simulink library "M160_lib"  (Simulink 7.8)
settings: Solver=FixedStepDiscrete  StartTime=0.0  StopTime=10.0  RelTol=1e-3
PreLoadFcn:
  | update_path
undefined symbols (not defined in the file): Afr_atCool2facLambdaReqCorr_CUR_x, Afr_atCool2facLambdaReqCorr_CUR_y, Afr_atMani2facLambdaReqCorr_CUR_x, Afr_atMani2facLambdaReqCorr_CUR_y, Afr_facLambdaReqMan, Afr_facRatioMan, Afr_facStoich, Afr_flgLambdaReqOverride, Afr_flgRatioOverride, Afr_rpmEngSpdfacRelAir2facLambdaReqBase_MAP_x, Afr_rpmEngSpdfacRelAir2facLambdaReqBase_MAP_y, Afr_rpmEngSpdfacRelAir2facLambdaReqBase_MAP_z, Ais_flgAirInjReacPumpOverride, Ais_stAirInjReacPumpMan, Amc_flgAirMassFlowOverride, Amc_uSens2AirMassFlow_CUR_x, Amc_uSens2AirMassFlow_CUR_y, Amc_uSensMaxValid, Amc_uSensMinValid, Amf_facRelAirMan, Amf_flgAirMassPerStrOverride, Amf_flgRelAirOverride, Amf_flgSwitch2AirMassFlowMeter, Amf_mAirPerStrMan, Amf_pManiEngSpd2facRelAirCorr_MAP_x, Amf_pManiEngSpd2facRelAirCorr_MAP_y, Amf_pManiEngSpd2facRelAirCorr_MAP_z, Amf_rpmEngSpd2facTempCorr_CUR_x, Amf_rpmEngSpd2facTempCorr_CUR_y, Amf_shcSpecGasConst_C, Amf_volEngDisp_C, Apv_facAirPumpRateMan, Apv_factor, Apv_flgAirPumpRateOverride, Apv_tiPeriod_C, Bvc_rVoltDivHigh, Bvc_rVoltDivLow, Bvc_uBattMax, Bvc_uBattMin, CDRV_E_OK_, Cov_facChOverVlvRateMan, Cov_factor, Cov_flgChOverVlvRateOverride, Cov_tiPeriod_C, Cpc_atManiTmp2facPresCorr_CUR_x, Cpc_atManiTmp2facPresCorr_CUR_y, Cpc_flgPChargeOverride, Cpc_uSens2pManiBase_CUR_x, Cpc_uSens2pManiBase_CUR_y, Ctc_rPullUp_C, Ctc_rSens2atCool_CUR_x, Ctc_rSens2atCool_CUR_y, Ctc_uSensMaxValid, Ctc_uSensMinValid, Ctc_uSupply, Doh_OutputDiagnosisOverride, dummy_facAirPumpRateReq, dummy_facChOverVlvRateReq, dummy_flgInterCoolerOverride, dummy_flgKl50Override ... (+243)
libraries: simulink x36, ehooks_lib x3
(part 6 of 8)

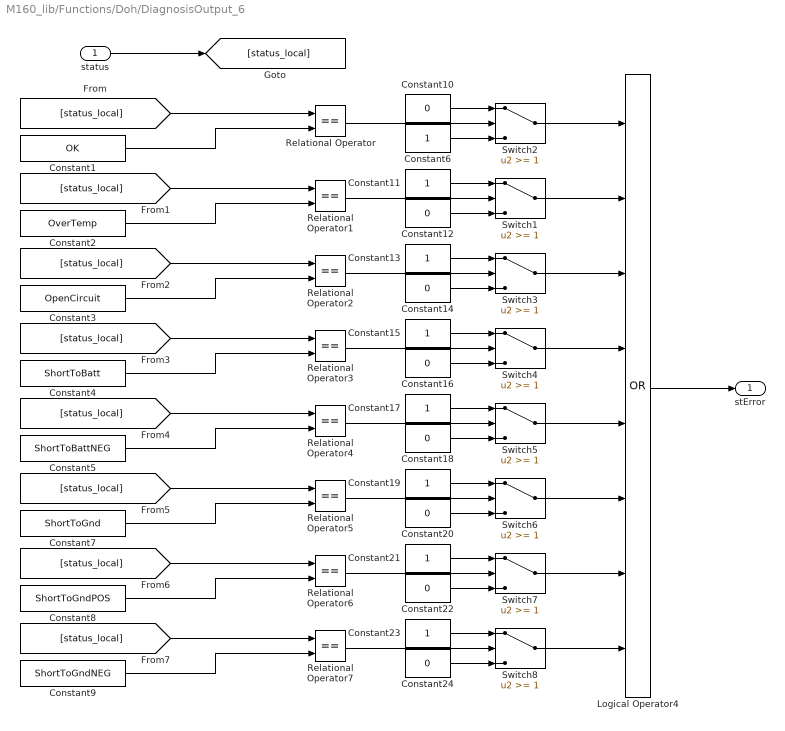
== system M160_lib/Functions/Doh/DiagnosisOutput_6 ==
  status : Inport
  Constant1 : Constant  Value=OK
  Constant{10,12,14,16,18,20,22,24} (8 alike) : Constant  Value=0  OutDataTypeStr=boolean
  Constant{6,11,13,15,17,19,21,23} (8 alike) : Constant  OutDataTypeStr=boolean
  Constant2 : Constant  Value=OverTemp
  Constant3 : Constant  Value=OpenCircuit
  Constant4 : Constant  Value=ShortToBatt
  Constant5 : Constant  Value=ShortToBattNEG
  Constant7 : Constant  Value=ShortToGnd
  Constant8 : Constant  Value=ShortToGndPOS
  Constant9 : Constant  Value=ShortToGndNEG
  Logical Operator4 : Logic  Operator=OR  Inputs=8  AllPortsSameDT=off  OutDataTypeStr=boolean
  Relational Operator{,1..7} (8 alike) : RelationalOperator  Operator===  OutDataTypeStr=boolean
  Switch{1..8} (8 alike) : Switch  Threshold=1
  stError : Outport
  wires:
  Switch8/1 -> Logical Operator4/8
  Switch7/1 -> Logical Operator4/7
  Switch6/1 -> Logical Operator4/6
  Switch5/1 -> Logical Operator4/5
  Switch4/1 -> Logical Operator4/4
  Switch3/1 -> Logical Operator4/3
  Switch1/1 -> Logical Operator4/2
  Switch2/1 -> Logical Operator4/1
  Relational Operator7/1 -> Switch8/2
  Constant23/1 -> Switch8/1
  Constant24/1 -> Switch8/3
  Relational Operator6/1 -> Switch7/2
  Constant21/1 -> Switch7/1
  Constant22/1 -> Switch7/3
  Relational Operator5/1 -> Switch6/2
  Constant19/1 -> Switch6/1
  Constant20/1 -> Switch6/3
  Relational Operator4/1 -> Switch5/2
  Constant17/1 -> Switch5/1
  Constant18/1 -> Switch5/3
  Relational Operator3/1 -> Switch4/2
  Constant15/1 -> Switch4/1
  Constant16/1 -> Switch4/3
  Relational Operator2/1 -> Switch3/2
  Constant13/1 -> Switch3/1
  Constant14/1 -> Switch3/3
  Relational Operator1/1 -> Switch1/2
  Constant11/1 -> Switch1/1
  Constant12/1 -> Switch1/3
  Constant10/1 -> Switch2/1
  Logical Operator4/1 -> stError/1
  Constant6/1 -> Switch2/3
  Relational Operator/1 -> Switch2/2
  [status_local] -> Relational Operator7/1
  Constant9/1 -> Relational Operator7/2
  [status_local] -> Relational Operator6/1
  Constant8/1 -> Relational Operator6/2
  [status_local] -> Relational Operator5/1
  Constant7/1 -> Relational Operator5/2
  [status_local] -> Relational Operator4/1
  Constant5/1 -> Relational Operator4/2
  [status_local] -> Relational Operator3/1
  Constant4/1 -> Relational Operator3/2
  [status_local] -> Relational Operator2/1
  Constant3/1 -> Relational Operator2/2
  [status_local] -> Relational Operator1/1
  Constant2/1 -> Relational Operator1/2
  [status_local] -> Relational Operator/1
  status/1 -> [status_local]
  Constant1/1 -> Relational Operator/2

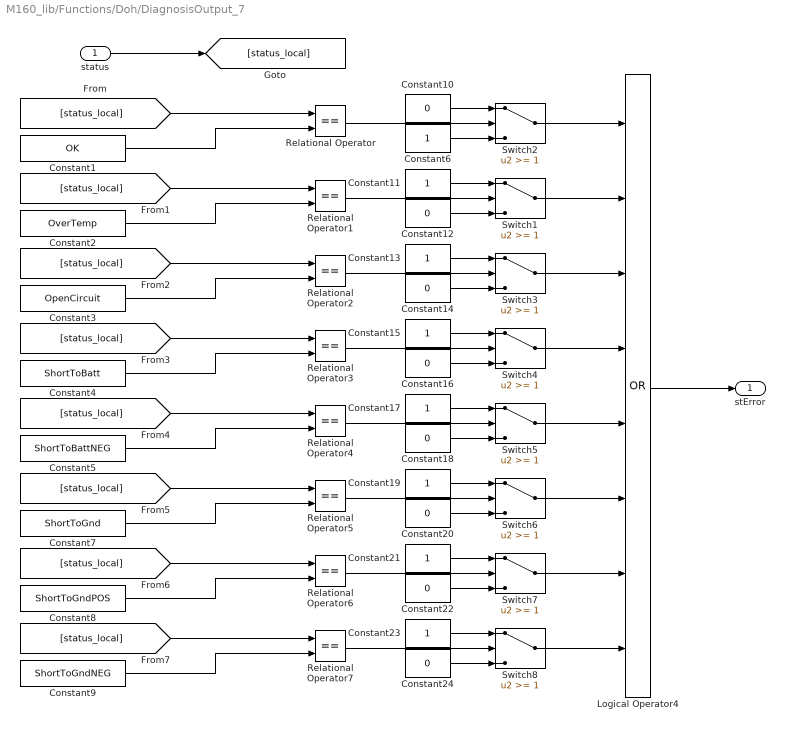
== system M160_lib/Functions/Doh/DiagnosisOutput_7 ==
  status : Inport
  Constant1 : Constant  Value=OK
  Constant{10,12,14,16,18,20,22,24} (8 alike) : Constant  Value=0  OutDataTypeStr=boolean
  Constant{6,11,13,15,17,19,21,23} (8 alike) : Constant  OutDataTypeStr=boolean
  Constant2 : Constant  Value=OverTemp
  Constant3 : Constant  Value=OpenCircuit
  Constant4 : Constant  Value=ShortToBatt
  Constant5 : Constant  Value=ShortToBattNEG
  Constant7 : Constant  Value=ShortToGnd
  Constant8 : Constant  Value=ShortToGndPOS
  Constant9 : Constant  Value=ShortToGndNEG
  Logical Operator4 : Logic  Operator=OR  Inputs=8  AllPortsSameDT=off  OutDataTypeStr=boolean
  Relational Operator{,1..7} (8 alike) : RelationalOperator  Operator===  OutDataTypeStr=boolean
  Switch{1..8} (8 alike) : Switch  Threshold=1
  stError : Outport
  wires:
  Constant1/1 -> Relational Operator/2
  status/1 -> [status_local]
  [status_local] -> Relational Operator/1
  Constant2/1 -> Relational Operator1/2
  [status_local] -> Relational Operator1/1
  Constant3/1 -> Relational Operator2/2
  [status_local] -> Relational Operator2/1
  Constant4/1 -> Relational Operator3/2
  [status_local] -> Relational Operator3/1
  Constant5/1 -> Relational Operator4/2
  [status_local] -> Relational Operator4/1
  Constant7/1 -> Relational Operator5/2
  [status_local] -> Relational Operator5/1
  Constant8/1 -> Relational Operator6/2
  [status_local] -> Relational Operator6/1
  Constant9/1 -> Relational Operator7/2
  [status_local] -> Relational Operator7/1
  Relational Operator/1 -> Switch2/2
  Constant6/1 -> Switch2/3
  Logical Operator4/1 -> stError/1
  Constant10/1 -> Switch2/1
  Constant12/1 -> Switch1/3
  Constant11/1 -> Switch1/1
  Relational Operator1/1 -> Switch1/2
  Constant14/1 -> Switch3/3
  Constant13/1 -> Switch3/1
  Relational Operator2/1 -> Switch3/2
  Constant16/1 -> Switch4/3
  Constant15/1 -> Switch4/1
  Relational Operator3/1 -> Switch4/2
  Constant18/1 -> Switch5/3
  Constant17/1 -> Switch5/1
  Relational Operator4/1 -> Switch5/2
  Constant20/1 -> Switch6/3
  Constant19/1 -> Switch6/1
  Relational Operator5/1 -> Switch6/2
  Constant22/1 -> Switch7/3
  Constant21/1 -> Switch7/1
  Relational Operator6/1 -> Switch7/2
  Constant24/1 -> Switch8/3
  Constant23/1 -> Switch8/1
  Relational Operator7/1 -> Switch8/2
  Switch2/1 -> Logical Operator4/1
  Switch1/1 -> Logical Operator4/2
  Switch3/1 -> Logical Operator4/3
  Switch4/1 -> Logical Operator4/4
  Switch5/1 -> Logical Operator4/5
  Switch6/1 -> Logical Operator4/6
  Switch7/1 -> Logical Operator4/7
  Switch8/1 -> Logical Operator4/8

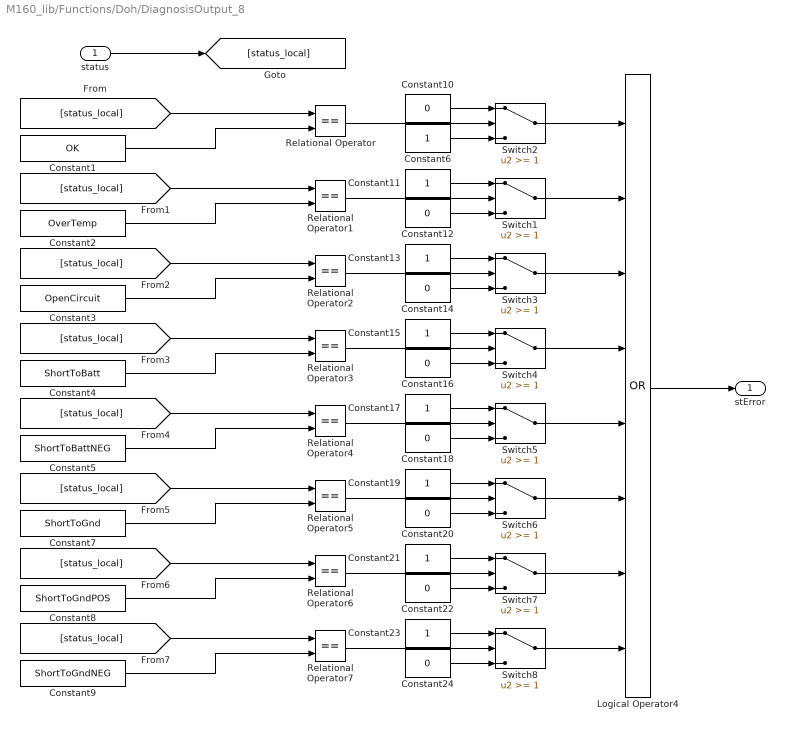
== system M160_lib/Functions/Doh/DiagnosisOutput_8 ==
  status : Inport
  Constant1 : Constant  Value=OK
  Constant{10,12,14,16,18,20,22,24} (8 alike) : Constant  Value=0  OutDataTypeStr=boolean
  Constant{6,11,13,15,17,19,21,23} (8 alike) : Constant  OutDataTypeStr=boolean
  Constant2 : Constant  Value=OverTemp
  Constant3 : Constant  Value=OpenCircuit
  Constant4 : Constant  Value=ShortToBatt
  Constant5 : Constant  Value=ShortToBattNEG
  Constant7 : Constant  Value=ShortToGnd
  Constant8 : Constant  Value=ShortToGndPOS
  Constant9 : Constant  Value=ShortToGndNEG
  Logical Operator4 : Logic  Operator=OR  Inputs=8  AllPortsSameDT=off  OutDataTypeStr=boolean
  Relational Operator{,1..7} (8 alike) : RelationalOperator  Operator===  OutDataTypeStr=boolean
  Switch{1..8} (8 alike) : Switch  Threshold=1
  stError : Outport
  wires:
  Switch8/1 -> Logical Operator4/8
  Switch7/1 -> Logical Operator4/7
  Switch6/1 -> Logical Operator4/6
  Switch5/1 -> Logical Operator4/5
  Switch4/1 -> Logical Operator4/4
  Switch3/1 -> Logical Operator4/3
  Switch1/1 -> Logical Operator4/2
  Switch2/1 -> Logical Operator4/1
  Relational Operator7/1 -> Switch8/2
  Constant23/1 -> Switch8/1
  Constant24/1 -> Switch8/3
  Relational Operator6/1 -> Switch7/2
  Constant21/1 -> Switch7/1
  Constant22/1 -> Switch7/3
  Relational Operator5/1 -> Switch6/2
  Constant19/1 -> Switch6/1
  Constant20/1 -> Switch6/3
  Relational Operator4/1 -> Switch5/2
  Constant17/1 -> Switch5/1
  Constant18/1 -> Switch5/3
  Relational Operator3/1 -> Switch4/2
  Constant15/1 -> Switch4/1
  Constant16/1 -> Switch4/3
  Relational Operator2/1 -> Switch3/2
  Constant13/1 -> Switch3/1
  Constant14/1 -> Switch3/3
  Relational Operator1/1 -> Switch1/2
  Constant11/1 -> Switch1/1
  Constant12/1 -> Switch1/3
  Constant10/1 -> Switch2/1
  Logical Operator4/1 -> stError/1
  Constant6/1 -> Switch2/3
  Relational Operator/1 -> Switch2/2
  [status_local] -> Relational Operator7/1
  Constant9/1 -> Relational Operator7/2
  [status_local] -> Relational Operator6/1
  Constant8/1 -> Relational Operator6/2
  [status_local] -> Relational Operator5/1
  Constant7/1 -> Relational Operator5/2
  [status_local] -> Relational Operator4/1
  Constant5/1 -> Relational Operator4/2
  [status_local] -> Relational Operator3/1
  Constant4/1 -> Relational Operator3/2
  [status_local] -> Relational Operator2/1
  Constant3/1 -> Relational Operator2/2
  [status_local] -> Relational Operator1/1
  Constant2/1 -> Relational Operator1/2
  [status_local] -> Relational Operator/1
  status/1 -> [status_local]
  Constant1/1 -> Relational Operator/2

== system M160_lib/Functions/Doh/DiagnosisOutput_9 ==
  status : Inport
  Constant1 : Constant  Value=OK
  Constant{10,12,14,16,18,20,22,24} (8 alike) : Constant  Value=0  OutDataTypeStr=boolean
  Constant{6,11,13,15,17,19,21,23} (8 alike) : Constant  OutDataTypeStr=boolean
  Constant2 : Constant  Value=OverTemp
  Constant3 : Constant  Value=OpenCircuit
  Constant4 : Constant  Value=ShortToBatt
  Constant5 : Constant  Value=ShortToBattNEG
  Constant7 : Constant  Value=ShortToGnd
  Constant8 : Constant  Value=ShortToGndPOS
  Constant9 : Constant  Value=ShortToGndNEG
  Logical Operator4 : Logic  Operator=OR  Inputs=8  AllPortsSameDT=off  OutDataTypeStr=boolean
  Relational Operator{,1..7} (8 alike) : RelationalOperator  Operator===  OutDataTypeStr=boolean
  Switch{1..8} (8 alike) : Switch  Threshold=1
  stError : Outport
  wires:
  Constant1/1 -> Relational Operator/2
  status/1 -> [status_local]
  [status_local] -> Relational Operator/1
  Constant2/1 -> Relational Operator1/2
  [status_local] -> Relational Operator1/1
  Constant3/1 -> Relational Operator2/2
  [status_local] -> Relational Operator2/1
  Constant4/1 -> Relational Operator3/2
  [status_local] -> Relational Operator3/1
  Constant5/1 -> Relational Operator4/2
  [status_local] -> Relational Operator4/1
  Constant7/1 -> Relational Operator5/2
  [status_local] -> Relational Operator5/1
  Constant8/1 -> Relational Operator6/2
  [status_local] -> Relational Operator6/1
  Constant9/1 -> Relational Operator7/2
  [status_local] -> Relational Operator7/1
  Relational Operator/1 -> Switch2/2
  Constant6/1 -> Switch2/3
  Logical Operator4/1 -> stError/1
  Constant10/1 -> Switch2/1
  Constant12/1 -> Switch1/3
  Constant11/1 -> Switch1/1
  Relational Operator1/1 -> Switch1/2
  Constant14/1 -> Switch3/3
  Constant13/1 -> Switch3/1
  Relational Operator2/1 -> Switch3/2
  Constant16/1 -> Switch4/3
  Constant15/1 -> Switch4/1
  Relational Operator3/1 -> Switch4/2
  Constant18/1 -> Switch5/3
  Constant17/1 -> Switch5/1
  Relational Operator4/1 -> Switch5/2
  Constant20/1 -> Switch6/3
  Constant19/1 -> Switch6/1
  Relational Operator5/1 -> Switch6/2
  Constant22/1 -> Switch7/3
  Constant21/1 -> Switch7/1
  Relational Operator6/1 -> Switch7/2
  Constant24/1 -> Switch8/3
  Constant23/1 -> Switch8/1
  Relational Operator7/1 -> Switch8/2
  Switch2/1 -> Logical Operator4/1
  Switch1/1 -> Logical Operator4/2
  Switch3/1 -> Logical Operator4/3
  Switch4/1 -> Logical Operator4/4
  Switch5/1 -> Logical Operator4/5
  Switch6/1 -> Logical Operator4/6
  Switch7/1 -> Logical Operator4/7
  Switch8/1 -> Logical Operator4/8

== system M160_lib/Functions/Fmc/DT1 ==
  T : Inport
  K : Inport  Port=2
  Ta : Inport  Port=3
  in : Inport  Port=4
  initValue : Inport  Port=5
  Enable : Inport  Port=6
  Add2 : Sum  OutDataTypeStr=Inherit: Same as first input
  Constan3 : Constant  OutDataTypeStr=single
  Divide1 : Product  Inputs=*/  OutDataTypeStr=Inherit: Same as first input
  Product1 : Product  Inputs=3  OutDataTypeStr=Inherit: Same as first input
  Product3 : Product  OutDataTypeStr=Inherit: Same as first input
  Product4 : Product  OutDataTypeStr=Inherit: Same as first input
  Subtract1 : Sum  Inputs=+-
  Switch1 : Switch  Threshold=1
  Unit Delay4 : UnitDelay  SampleTime=-1
  Unit Delay5 : UnitDelay  SampleTime=-1
  Unit Delay6 : UnitDelay  SampleTime=-1
  Out : Outport
  wires:
  initValue/1 -> Switch1/3
  Switch1/1 -> Out/1
  in/1 -> Subtract1/1
  Subtract1/1 -> Product3/2
  K/1 -> Product3/1, Product4/2
  Product3/1 -> Unit Delay6/1
  Unit Delay6/1 -> Product1/1
  Constan3/1 -> Divide1/1
  T/1 -> Product4/1
  Product4/1 -> Divide1/2
  Divide1/1 -> Product1/2
  Product1/1 -> Add2/1
  Add2/1 -> Unit Delay5/1, Unit Delay4/1, Switch1/1
  Unit Delay5/1 -> Add2/2
  Unit Delay4/1 -> Subtract1/2
  Ta/1 -> Product1/3
  Enable/1 -> Switch1/2

== system M160_lib/Functions/Fmc/DT1_Fcn ==
  In : Inport
  initValue : Inport  Port=2
  Enable : Inport  Port=3
  Discrete Transfer Fcn : DiscreteTransferFcn  Numerator=[Fmc_facKFuelMassCorr Fmc_facKFuelMassCorr*(0.001/Fmc_tiTFuelMassCorr-1)]  Denominator=[1 -1]  SampleTime=-1  OutDataTypeStr=Inherit: Same as input
  Switch1 : Switch  Threshold=1
  Out : Outport
  wires:
  In/1 -> Discrete Transfer Fcn/1
  initValue/1 -> Switch1/3
  Switch1/1 -> Out/1
  Discrete Transfer Fcn/1 -> Switch1/1
  Enable/1 -> Switch1/2

== system M160_lib/Functions/ICC_1/RSFlipFlop ==
  s : Inport
  r : Inport  Port=2
  Gain : Gain  OutDataTypeStr=Inherit: Same as input
  Logical Operator3 : Logic  Operator=NOT  AllPortsSameDT=off  OutDataTypeStr=boolean
  MATLAB Function : MATLAB Function  TreatAsAtomicUnit=on
  Unit Delay : UnitDelay  SampleTime=-1
  q : Outport
  nq : Outport  Port=2
  wires:
  Logical Operator3/1 -> nq/1
  r/1 -> MATLAB Function/1(r)
  s/1 -> MATLAB Function/2(s)
  MATLAB Function/1(q) -> Unit Delay/1
  Gain/1 -> q/1
  Unit Delay/1 -> Logical Operator3/1, Gain/1

== system M160_lib/Functions/Isc/CounterEnabled ==
  initEnable : Inport
  enable : Inport  Port=2
  Add1 : Sum
  Constant1 : Constant  OutDataTypeStr=single
  Constant2 : Constant  Value=0  OutDataTypeStr=single
  MATLAB Function : MATLAB Function  TreatAsAtomicUnit=on
  Switch2 : Switch  Threshold=1
  Unit Delay : UnitDelay  SampleTime=-1
  Unit Delay1 : UnitDelay  SampleTime=-1
  return : Outport
  wires:
  initEnable/1 -> MATLAB Function/1(u)
  MATLAB Function/1(y) -> Switch2/2
  Add1/1 -> Unit Delay1/1, Switch2/1
  Constant2/1 -> Switch2/3
  Switch2/1 -> Unit Delay/1
  Unit Delay1/1 -> Add1/2
  Constant1/1 -> Add1/1
  enable/1 -> MATLAB Function/2(v)
  Unit Delay/1 -> return/1

== system M160_lib/Functions/Isc/EdgeFalling ==
  signal : Inport
  Detect Decrease : simulink/Logic and Bit Operations/Detect Decrease  vinit=0.0  InputProcessing=Inherited  OutDataTypeStr=boolean
  return : Outport
  wires:
  Detect Decrease/1 -> return/1
  signal/1 -> Detect Decrease/1

== system M160_lib/Functions/Isc/EdgeRising ==
  signal : Inport
  Detect Increase : simulink/Logic and Bit Operations/Detect Increase  vinit=0.0  InputProcessing=Inherited  OutDataTypeStr=boolean
  return : Outport
  wires:
  Detect Increase/1 -> return/1
  signal/1 -> Detect Increase/1

== system M160_lib/Functions/Isc/Integrator ==
  initEnable : Inport
  enable : Inport  Port=2
  in : Inport  Port=3
  deltaT : Inport  Port=4
  mx : Inport  Port=5
  mn : Inport  Port=6
  initValue : Inport  Port=7
  Add : Sum
  MATLAB Function : MATLAB Function  TreatAsAtomicUnit=on
  MinMax : MinMax  Function=max  Inputs=2
  MinMax1 : MinMax  Inputs=2
  Product1 : Product  OutDataTypeStr=Inherit: Same as first input
  Unit Delay : UnitDelay  SampleTime=-1
  Unit Delay1 : UnitDelay  SampleTime=-1
  return : Outport
  wires:
  deltaT/1 -> Product1/2
  in/1 -> Product1/1
  Product1/1 -> Add/1
  Add/1 -> MinMax1/1
  mx/1 -> MinMax1/2
  MinMax1/1 -> MinMax/1
  mn/1 -> MinMax/2
  Unit Delay/1 -> Add/2
  MinMax/1 -> Unit Delay/1, MATLAB Function/4(in)
  MATLAB Function/1(out) -> Unit Delay1/1
  enable/1 -> MATLAB Function/3(enable)
  initValue/1 -> MATLAB Function/2(initValue)
  initEnable/1 -> MATLAB Function/1(initEnable)
  Unit Delay1/1 -> return/1

== system M160_lib/Functions/Isc/Integrator1 ==
  initEnable : Inport
  enable : Inport  Port=2
  in : Inport  Port=3
  deltaT : Inport  Port=4
  mx : Inport  Port=5
  mn : Inport  Port=6
  initValue : Inport  Port=7
  Add : Sum
  MATLAB Function : MATLAB Function  TreatAsAtomicUnit=on
  MinMax : MinMax  Function=max  Inputs=2
  MinMax1 : MinMax  Inputs=2
  Product1 : Product  OutDataTypeStr=Inherit: Same as first input
  Unit Delay : UnitDelay  SampleTime=-1
  Unit Delay1 : UnitDelay  SampleTime=-1
  return : Outport
  wires:
  Unit Delay1/1 -> return/1
  initEnable/1 -> MATLAB Function/1(initEnable)
  initValue/1 -> MATLAB Function/2(initValue)
  enable/1 -> MATLAB Function/3(enable)
  MATLAB Function/1(out) -> Unit Delay1/1
  MinMax/1 -> MATLAB Function/4(in), Unit Delay/1
  Unit Delay/1 -> Add/2
  mn/1 -> MinMax/2
  MinMax1/1 -> MinMax/1
  mx/1 -> MinMax1/2
  Add/1 -> MinMax1/1
  Product1/1 -> Add/1
  in/1 -> Product1/1
  deltaT/1 -> Product1/2

== system M160_lib/Functions/Itc/Hysteresis_Delta_RSP ==
  in : Inport
  Relay : Relay  OnSwitchValue=Itc_rpmEngSpdMax  OffSwitchValue=Itc_rpmEngSpdMax-Itc_rpmEngSpdHyst  OutDataTypeStr=Inherit: Inherit via back propagation
  return : Outport
  wires:
  Relay/1 -> return/1
  in/1 -> Relay/1

== system M160_lib/Functions/Lcc/PID-Controller ==
  in : Inport
  Lcc_flgSwitch2PIDController : Inport  Port=2
  dt : Inport  Port=3
  Lamsoni : Inport  Port=4
  Afr_facLambdaReq : Inport  Port=5
  Epm_rpmEngSpd : Inport  Port=6
  Mpc_pManiFilt : Inport  Port=7
  Constant8 : Constant  Value=Lcc_LambdaCorrMaxPID
  Constant9 : Constant  Value=Lcc_LambdaCorrMinPID
  Lcc_facKLambdaCorrPID_MAP : Lookup_n-D  BreakpointsForDimension1=Lcc_facKLambdaCorrPID_MAP_x  BreakpointsForDimension2=Lcc_facKLambdaCorrPID_MAP_y  Table=Lcc_facKLambdaCorrPID_MAP_z  ExtrapMethod=Clip  InputSameDT=on
  Lcc_tiTnLambdaCorrPID_MAP : Lookup_n-D  BreakpointsForDimension1=Lcc_tiTnLambdaCorrPID_MAP_x  BreakpointsForDimension2=Lcc_tiTnLambdaCorrPID_MAP_y  Table=Lcc_tiTnLambdaCorrPID_MAP_z  ExtrapMethod=Clip  InputSameDT=on
  Lcc_tiTvLambdaCorrPID_MAP : Lookup_n-D  BreakpointsForDimension1=Lcc_tiTvLambdaCorrPID_MAP_x  BreakpointsForDimension2=Lcc_tiTvLambdaCorrPID_MAP_y  Table=Lcc_tiTvLambdaCorrPID_MAP_z  ExtrapMethod=Clip  InputSameDT=on
  Logical Operator2 : Logic  AllPortsSameDT=off  OutDataTypeStr=boolean
  PID_Limit_AWU : Subsystem
      mask Description: PID_Limit_AWU
      mask Display: image(imread('PID_Limit_AWU.jpg'))
  Subtract : Sum  Inputs=+-  OutDataTypeStr=Inherit: Same as first input
  Lcc_facLambdaPIDController : Outport
  wires:
  PID_Limit_AWU/1(Lcc_facLambdaPIDController) -> Lcc_facLambdaPIDController/1
  Epm_rpmEngSpd/1 -> Lcc_tiTnLambdaCorrPID_MAP/1, Lcc_tiTvLambdaCorrPID_MAP/1, Lcc_facKLambdaCorrPID_MAP/1
  Mpc_pManiFilt/1 -> Lcc_tiTnLambdaCorrPID_MAP/2, Lcc_tiTvLambdaCorrPID_MAP/2, Lcc_facKLambdaCorrPID_MAP/2
  Lcc_tiTnLambdaCorrPID_MAP/1 -> PID_Limit_AWU/1(Tn)
  Lcc_tiTvLambdaCorrPID_MAP/1 -> PID_Limit_AWU/2(Tv)
  dt/1 -> PID_Limit_AWU/3(Ta)
  Lcc_facKLambdaCorrPID_MAP/1 -> PID_Limit_AWU/4(Kp)
  Subtract/1 -> PID_Limit_AWU/5(in)
  Constant8/1 -> PID_Limit_AWU/7(outMax)
  Constant9/1 -> PID_Limit_AWU/8(outMin)
  Lamsoni/1 -> Subtract/1
  Afr_facLambdaReq/1 -> Subtract/2
  in/1 -> Logical Operator2/1
  Lcc_flgSwitch2PIDController/1 -> Logical Operator2/2
  Logical Operator2/1 -> PID_Limit_AWU/6(initValue)

== system M160_lib/Functions/Lcc/Two-point-controller ==
  Lcc_flgSwitch2PIDController : Inport
  in : Inport  Port=2
  in1 : Inport  Port=3
  Epm_rpmEngSpd : Inport  Port=4
  dt : Inport  Port=5
  Constan1 : Constant  Value=-1  OutDataTypeStr=single
  Constan2 : Constant  Value=-1  OutDataTypeStr=single
  Constan3 : Constant  Value=0.0  OutDataTypeStr=single
  Constan8 : Constant  Value=0.0  OutDataTypeStr=single
  Constant1 : Constant  Value=Lcc_LambdaCorrMaxTPC
  Constant2 : Constant  Value=Lcc_LambdaCorrMinTPC
  Constant3 : Constant  Value=Lcc_facInitValue
  Constant4 : Constant  Value=Lcc_IntStartValueTPC
  EdgeFalling : Subsystem
      mask Description: EdgeFalling
      mask Display: image(imread('EdgeFalling.jpg'))
  EdgeFalling1 : Subsystem
      mask Description: EdgeFalling
      mask Display: image(imread('EdgeFalling.jpg'))
  EdgeRising : Subsystem
      mask Description: EdgeRising
      mask Display: image(imread('EdgeRising.jpg'))
  EdgeRising1 : Subsystem
      mask Description: EdgeRising
      mask Display: image(imread('EdgeRising.jpg'))
  Integrator : Subsystem
      mask Description: Integrator
      mask Display: image(imread('Integrator.jpg'))
  Lcc_EngSpd2facIntegrator_CUR : Lookup_n-D  NumberOfTableDimensions=1  BreakpointsForDimension1=Lcc_EngSpd2facIntegrator_CUR_x  Table=Lcc_EngSpd2facIntegrator_CUR_y  ExtrapMethod=Clip  InputSameDT=on
  Logical Operator1 : Logic  Operator=OR  AllPortsSameDT=off  OutDataTypeStr=boolean
  Logical Operator2 : Logic  Operator=OR  AllPortsSameDT=off  OutDataTypeStr=boolean
  Logical Operator3 : Logic  Operator=NOT  AllPortsSameDT=off  OutDataTypeStr=boolean
  Product1 : Product  OutDataTypeStr=Inherit: Same as first input
  Product2 : Product  OutDataTypeStr=Inherit: Same as first input
  Subtract1 : Sum  OutDataTypeStr=Inherit: Same as first input
  Switch{1..5} (5 alike) : Switch  Threshold=1
  Lcc_facLambdaTPCCorr : Outport
  wires:
  EdgeFalling/1(return) -> Logical Operator2/1
  EdgeRising/1(return) -> Logical Operator2/2
  in1/1 -> EdgeFalling/1(signal), EdgeRising/1(signal), Switch2/2, Switch4/2
  EdgeRising1/1(return) -> Logical Operator1/1
  EdgeFalling1/1(return) -> Logical Operator1/2
  in/1 -> Logical Operator3/1, Integrator/2(enable), EdgeRising1/1(signal)
  Logical Operator3/1 -> Switch1/2, Switch3/2
  Epm_rpmEngSpd/1 -> Lcc_EngSpd2facIntegrator_CUR/1
  Lcc_EngSpd2facIntegrator_CUR/1 -> Switch1/3, Product1/1
  Constan8/1 -> Switch1/1
  Switch1/1 -> Switch2/3
  Product1/1 -> Switch2/1
  Constan1/1 -> Product1/2
  Constant3/1 -> Product2/1, Switch3/3
  Switch3/1 -> Switch4/3
  Product2/1 -> Switch4/1
  Constan2/1 -> Product2/2
  Constan3/1 -> Switch3/1
  Switch4/1 -> Subtract1/1
  Logical Operator1/1 -> Switch5/2
  Subtract1/1 -> Switch5/3
  Constant4/1 -> Switch5/1
  Integrator/1(return) -> Lcc_facLambdaTPCCorr/1, Subtract1/2
  Logical Operator2/1 -> Integrator/1(initEnable)
  Switch2/1 -> Integrator/3(in)
  dt/1 -> Integrator/4(deltaT)
  Switch5/1 -> Integrator/7(initValue)  "Lcc_IntInitValvue"
  Constant1/1 -> Integrator/5(mx)
  Constant2/1 -> Integrator/6(mn)
  Lcc_flgSwitch2PIDController/1 -> EdgeFalling1/1(signal)

== system M160_lib/Functions/Opm/ErrorCheck ==
  Eih_flgInputError : Inport
  Doh_flgErrorDiagnosis : Inport  Port=2
  Eoh_flgOutputError : Inport  Port=3
  Opm_flgInputErrorMem : Inport  Port=4
  Opm_flgOutputErrorMem : Inport  Port=5
  function : TriggerPort  TriggerType=function-call
  Constant1 : Constant  Value=Opm_stIOErrorOverride
  Constant{3..4,6,9..11} (6 alike) : Constant  Value=0  OutDataTypeStr=boolean
  Constant2 : Constant  Value=Opm_stDiagnosisOverride
  Constant5 : Constant  Value=Opm_tiIOErrorDelay
  Constant7 : Constant  Value=1000  OutDataTypeStr=single
  Constant8 : Constant  Value=Opm_stEngControl
  Counter : Subsystem
      mask Description: Counter
      mask Display: image(imread('Counter.jpg'))
  Counter1 : Subsystem
      mask Description: Counter
      mask Display: image(imread('Counter.jpg'))
  Counter2 : Subsystem
      mask Description: Counter
      mask Display: image(imread('Counter.jpg'))
  Logical Operator : Logic  Operator=OR  AllPortsSameDT=off  OutDataTypeStr=boolean
  Logical Operator1 : Logic  Operator=OR  AllPortsSameDT=off  OutDataTypeStr=boolean
  Logical Operator2 : Logic  Operator=OR  AllPortsSameDT=off  OutDataTypeStr=boolean
  Logical Operator3 : Logic  Operator=OR  Inputs=3  AllPortsSameDT=off  OutDataTypeStr=boolean
  Logical Operator4 : Logic  Operator=OR  Inputs=3  AllPortsSameDT=off  OutDataTypeStr=boolean
  Product1 : Product  OutDataTypeStr=Inherit: Same as first input
  Relational Oprator : RelationalOperator  Operator=>  OutDataTypeStr=boolean
  Relational Oprator1 : RelationalOperator  Operator=>  OutDataTypeStr=boolean
  Relational Oprator2 : RelationalOperator  Operator=>  OutDataTypeStr=boolean
  Switch{1..6} (6 alike) : Switch  Threshold=1
  Unit Delay1 : UnitDelay  SampleTime=-1
  Unit Delay2 : UnitDelay  SampleTime=-1
  Unit Delay3 : UnitDelay  SampleTime=-1
  Opm_stEngControl : Outport
  Erh_flgIOErrorAct : Outport  Port=2
  Opm_flgIOErrorMemIn : Outport  Port=3
  wires:
  Constant6/1 -> Switch2/1
  Constant1/1 -> Switch2/2, Switch1/2, Switch3/2
  Eih_flgInputError/1 -> Switch2/3
  Constant3/1 -> Switch1/1
  Constant4/1 -> Switch3/1
  Doh_flgErrorDiagnosis/1 -> Switch3/3
  Eoh_flgOutputError/1 -> Switch1/3
  Switch3/1 -> Switch4/3
  Constant9/1 -> Switch4/1
  Constant2/1 -> Switch4/2
  Switch2/1 -> Counter/1(in), Logical Operator3/1
  Switch1/1 -> Counter1/1(in), Logical Operator3/2
  Switch4/1 -> Counter2/1(in), Logical Operator3/3
  Constant5/1 -> Product1/1
  Constant7/1 -> Product1/2
  Counter/1(Out1) -> Relational Oprator/1
  Counter1/1(Out1) -> Relational Oprator1/1
  Product1/1 -> Relational Oprator/2, Relational Oprator1/2, Relational Oprator2/2
  Counter2/1(Out1) -> Relational Oprator2/1
  Relational Oprator/1 -> Logical Operator1/1
  Relational Oprator1/1 -> Logical Operator/1
  Relational Oprator2/1 -> Logical Operator2/1
  Logical Operator1/1 -> Unit Delay3/1, Switch5/3  "Opm_flgInputErrorMem"
  Unit Delay3/1 -> Logical Operator1/2
  Unit Delay2/1 -> Logical Operator/2
  Logical Operator/1 -> Unit Delay2/1, Switch6/3  "Opm_flgOutputErrorMem"
  Unit Delay1/1 -> Logical Operator2/2
  Logical Operator2/1 -> Unit Delay1/1, Logical Operator4/3  "Opm_flgOutputDiagnosisErrorMem"
  Logical Operator3/1 -> Erh_flgIOErrorAct/1  "Opm_flgIOErrorAct"
  Constant8/1 -> Opm_stEngControl/1
  Logical Operator4/1 -> Opm_flgIOErrorMemIn/1
  Constant11/1 -> Switch5/1
  Constant10/1 -> Switch6/1
  Opm_flgInputErrorMem/1 -> Switch5/2
  Opm_flgOutputErrorMem/1 -> Switch6/2
  Switch5/1 -> Logical Operator4/1
  Switch6/1 -> Logical Operator4/2

== system M160_lib/Functions/Opm/OpMode ==
  Opm_stEngControl : Inport
  Erh_flgIOErrorAct : Inport  Port=2
  Opm_flgIOErrorMemIn : Inport  Port=3
  function : TriggerPort  TriggerType=function-call
  EdgeRising : Subsystem
      mask Description: EdgeRising
      mask Display: image(imread('EdgeRising.jpg'))
  Gain : Gain
  fcn_OpMode : MATLAB Function  TreatAsAtomicUnit=on
  Opm_idxMode : Outport
  Opm_flgInputErrorMem : Outport  Port=2
  Opm_flgOutputErrorMem : Outport  Port=3
  wires:
  Opm_stEngControl/1 -> fcn_OpMode/1(Opm_stEngControl)
  Erh_flgIOErrorAct/1 -> fcn_OpMode/2(Opm_flgIOErrorAct)
  Opm_flgIOErrorMemIn/1 -> fcn_OpMode/3(Opm_flgIOErrorMemIn)
  fcn_OpMode/1(Opm_idxAct) -> Gain/1
  fcn_OpMode/2(Opm_flgIOErrorReset) -> EdgeRising/1(signal)
  Gain/1 -> Opm_idxMode/1  "Opm_idxMode"
  EdgeRising/1(return) -> Opm_flgInputErrorMem/1, Opm_flgOutputErrorMem/1

== system M160_lib/Functions/Opm/Opm_ErrorCheck ==
  ECU_FcnCallTrigger_Source_DownStream : Subsystem  TreatAsAtomicUnit=on
  TriggerOut : Outport
  wires:
  ECU_FcnCallTrigger_Source_DownStream/1(TriggerOut) -> TriggerOut/1

== system M160_lib/Functions/Opm/Opm_set ==
  ECU_FcnCallTrigger_Source_DownStream : Subsystem  TreatAsAtomicUnit=on
  TriggerOut : Outport
  wires:
  ECU_FcnCallTrigger_Source_DownStream/1(TriggerOut) -> TriggerOut/1

== system M160_lib/Functions/Stc/CounterEnabled ==
  initEnable : Inport
  enable : Inport  Port=2
  Add1 : Sum
  Constant1 : Constant  OutDataTypeStr=single
  Constant2 : Constant  Value=0  OutDataTypeStr=single
  MATLAB Function : MATLAB Function  TreatAsAtomicUnit=on
  Switch2 : Switch  Threshold=1
  Unit Delay : UnitDelay  SampleTime=-1
  Unit Delay1 : UnitDelay  SampleTime=-1
  return : Outport
  wires:
  initEnable/1 -> MATLAB Function/1(u)
  MATLAB Function/1(y) -> Switch2/2
  Add1/1 -> Unit Delay1/1, Switch2/1
  Constant2/1 -> Switch2/3
  Switch2/1 -> Unit Delay/1
  Unit Delay1/1 -> Add1/2
  Constant1/1 -> Add1/1
  enable/1 -> MATLAB Function/2(v)
  Unit Delay/1 -> return/1

== system M160_lib/Functions/Stc/CounterEnabled1 ==
  initEnable : Inport
  enable : Inport  Port=2
  Add1 : Sum
  Constant1 : Constant  OutDataTypeStr=single
  Constant2 : Constant  Value=0  OutDataTypeStr=single
  MATLAB Function : MATLAB Function  TreatAsAtomicUnit=on
  Switch2 : Switch  Threshold=1
  Unit Delay : UnitDelay  SampleTime=-1
  Unit Delay1 : UnitDelay  SampleTime=-1
  return : Outport
  wires:
  enable/1 -> MATLAB Function/2(v)
  Constant1/1 -> Add1/1
  Unit Delay1/1 -> Add1/2
  Switch2/1 -> Unit Delay/1
  Constant2/1 -> Switch2/3
  Add1/1 -> Switch2/1, Unit Delay1/1
  MATLAB Function/1(y) -> Switch2/2
  initEnable/1 -> MATLAB Function/1(u)
  Unit Delay/1 -> return/1

== system M160_lib/Functions/Stc/RSFlipFlop ==
  s : Inport
  r : Inport  Port=2
  Gain : Gain  OutDataTypeStr=Inherit: Same as input
  Logical Operator3 : Logic  Operator=NOT  AllPortsSameDT=off  OutDataTypeStr=boolean
  MATLAB Function : MATLAB Function  TreatAsAtomicUnit=on
  Unit Delay : UnitDelay  SampleTime=-1
  q : Outport
  nq : Outport  Port=2
  wires:
  MATLAB Function/1(q) -> Unit Delay/1
  s/1 -> MATLAB Function/2(s)
  r/1 -> MATLAB Function/1(r)
  Logical Operator3/1 -> nq/1
  Unit Delay/1 -> Logical Operator3/1, Gain/1
  Gain/1 -> q/1

== system M160_lib/Functions/Stc/RSFlipFlop1 ==
  s : Inport
  r : Inport  Port=2
  Gain : Gain  OutDataTypeStr=Inherit: Same as input
  Logical Operator3 : Logic  Operator=NOT  AllPortsSameDT=off  OutDataTypeStr=boolean
  MATLAB Function : MATLAB Function  TreatAsAtomicUnit=on
  Unit Delay : UnitDelay  SampleTime=-1
  q : Outport
  nq : Outport  Port=2
  wires:
  Logical Operator3/1 -> nq/1
  r/1 -> MATLAB Function/1(r)
  s/1 -> MATLAB Function/2(s)
  MATLAB Function/1(q) -> Unit Delay/1
  Unit Delay/1 -> Logical Operator3/1, Gain/1
  Gain/1 -> q/1

== system M160_lib/Functions/Stc/RSFlipFlop2 ==
  s : Inport
  r : Inport  Port=2
  Gain : Gain  OutDataTypeStr=Inherit: Same as input
  Logical Operator3 : Logic  Operator=NOT  AllPortsSameDT=off  OutDataTypeStr=boolean
  MATLAB Function : MATLAB Function  TreatAsAtomicUnit=on
  Unit Delay : UnitDelay  SampleTime=-1
  q : Outport
  nq : Outport  Port=2
  wires:
  MATLAB Function/1(q) -> Unit Delay/1
  s/1 -> MATLAB Function/2(s)
  r/1 -> MATLAB Function/1(r)
  Logical Operator3/1 -> nq/1
  Unit Delay/1 -> Logical Operator3/1, Gain/1
  Gain/1 -> q/1

== system M160_lib/Functions/Stc/RSFlipFlop3 ==
  s : Inport
  r : Inport  Port=2
  Gain : Gain  OutDataTypeStr=Inherit: Same as input
  Logical Operator3 : Logic  Operator=NOT  AllPortsSameDT=off  OutDataTypeStr=boolean
  MATLAB Function : MATLAB Function  TreatAsAtomicUnit=on
  Unit Delay : UnitDelay  SampleTime=-1
  q : Outport
  nq : Outport  Port=2
  wires:
  Logical Operator3/1 -> nq/1
  r/1 -> MATLAB Function/1(r)
  s/1 -> MATLAB Function/2(s)
  MATLAB Function/1(q) -> Unit Delay/1
  Unit Delay/1 -> Logical Operator3/1, Gain/1
  Gain/1 -> q/1

== system M160_lib/Functions/T2t/ThrottleValveControl ==
  Stc_flgStarterActive : Inport
  Epm_rpmEngSpd : Inport  Port=2
  T2t_pManiReqSlow : Inport  Port=3
  Mpc_pManiFilt : Inport  Port=4
  T2t_flgWasteGateControllerTrue : Inport  Port=5
  Constan1 : Constant  Value=40  OutDataTypeStr=single
  Constan2 : Constant  OutDataTypeStr=single
  Constan3 : Constant  Value=0  OutDataTypeStr=single
  Constant1 : Constant  Value=T2t_facThrValveReqCorrEnable
  Constant5 : Constant  Value=T2t_tiTnThrValveReqCorr
  Constant6 : Constant  Value=T2t_tiTvThrValveReqCorr
  Constant7 : Constant  Value=T2t_facKThrValveReqCorr
  Constant8 : Constant  Value=T2t_ThrValveReqCorrMax
  Constant9 : Constant  Value=T2t_ThrValveReqCorrMin
  Divide1 : Product  Inputs=*/  OutDataTypeStr=Inherit: Same as first input
  EdgeFalling : Subsystem
      mask Description: EdgeFalling
      mask Display: image(imread('EdgeFalling.jpg'))
  Logical Operator2 : Logic  Operator=OR  AllPortsSameDT=off  OutDataTypeStr=boolean
  MinMax : MinMax  Function=max  Inputs=2
  PID_Limit_AWU : Subsystem
      mask Description: PID_Limit_AWU
      mask Display: image(imread('PID_Limit_AWU.jpg'))
  Subtract : Sum  Inputs=+-  OutDataTypeStr=Inherit: Same as first input
  Subtract1 : Sum  OutDataTypeStr=Inherit: Same as first input
  Switch1 : Switch  Threshold=1
  T2t_rpmEngSpdpManiReq2facThrValveReqBase_MAP : Lookup_n-D  BreakpointsForDimension1=T2t_rpmEngSpdpManiReq2facThrValveReqBase_MAP_x  BreakpointsForDimension2=T2t_rpmEngSpdpManiReq2facThrValveReqBase_MAP_y  Table=T2t_rpmEngSpdpManiReq2facThrValveReqBase_MAP_z  ExtrapMethod=Clip  InputSameDT=on
  T2t_facThrValveReq : Outport
  wires:
  Constant5/1 -> PID_Limit_AWU/1(Tn)
  Subtract/1 -> PID_Limit_AWU/5(in)
  Constant6/1 -> PID_Limit_AWU/2(Tv)
  Constant7/1 -> PID_Limit_AWU/4(Kp)
  Constant8/1 -> PID_Limit_AWU/7(outMax)
  Constant9/1 -> PID_Limit_AWU/8(outMin)
  Epm_rpmEngSpd/1 -> T2t_rpmEngSpdpManiReq2facThrValveReqBase_MAP/1, MinMax/1
  T2t_pManiReqSlow/1 -> T2t_rpmEngSpdpManiReq2facThrValveReqBase_MAP/2, Subtract/1
  T2t_rpmEngSpdpManiReq2facThrValveReqBase_MAP/1 -> Subtract1/1  "T2t_facThrValveReqBase"
  Subtract1/1 -> T2t_facThrValveReq/1
  Constant1/1 -> Switch1/2
  Switch1/1 -> Subtract1/2
  Mpc_pManiFilt/1 -> Subtract/2
  T2t_flgWasteGateControllerTrue/1 -> Logical Operator2/1
  Stc_flgStarterActive/1 -> EdgeFalling/1(signal)
  EdgeFalling/1(return) -> Logical Operator2/2
  Logical Operator2/1 -> PID_Limit_AWU/6(initValue)
  Divide1/1 -> PID_Limit_AWU/3(Ta)  "T2t_tiTaThrValveReqCorr"
  Constan1/1 -> Divide1/1
  MinMax/1 -> Divide1/2
  Constan2/1 -> MinMax/2
  Constan3/1 -> Switch1/3
  PID_Limit_AWU/1(T2t_facThrValveReqCorr) -> Switch1/1  "T2t_facThrValveReqCorr"

== system M160_lib/Functions/T2t/WastegateControl ==
  Epm_rpmEngSpd : Inport
  T2t_pManiReqSlow : Inport  Port=2
  Mpc_pManiFilt : Inport  Port=3
  T2t_flgWasteGateControllerTrue : Inport  Port=4
  Constan1 : Constant  Value=40  OutDataTypeStr=single
  Constan2 : Constant  OutDataTypeStr=single
  Constant2 : Constant  Value=T2t_facWastegateReqCorrEnable
  Constant5 : Constant  Value=T2t_tiTnWastegateReqCorr
  Constant6 : Constant  Value=T2t_tiTvWastegateReqCorr
  Constant7 : Constant  Value=T2t_KWastegateReqCorr
  Constant8 : Constant
  Constant9 : Constant  Value=-1
  Divide1 : Product  Inputs=*/  OutDataTypeStr=Inherit: Same as first input
  Logical Operator2 : Logic  AllPortsSameDT=off  OutDataTypeStr=boolean
  MinMax : MinMax  Function=max  Inputs=2
  PID_Limit_AWU : Subsystem
      mask Description: PID_Limit_AWU
      mask Display: image(imread('PID_Limit_AWU.jpg'))
  Subtract : Sum  Inputs=+-  OutDataTypeStr=Inherit: Same as first input
  Subtract1 : Sum  OutDataTypeStr=Inherit: Same as first input
  T2t_rpmEngSpdpManiReq2facWastegateReqBase_MAP : Lookup_n-D  BreakpointsForDimension1=T2t_rpmEngSpdpManiReq2facWastegateReqBase_MAP_x  BreakpointsForDimension2=T2t_rpmEngSpdpManiReq2facWastegateReqBase_MAP_y  Table=T2t_rpmEngSpdpManiReq2facWastegateReqBase_MAP_z  ExtrapMethod=Clip  InputSameDT=on
  T2t_facWasteGateRate : Outport
  wires:
  Constan2/1 -> MinMax/2
  MinMax/1 -> Divide1/2
  Constan1/1 -> Divide1/1
  Divide1/1 -> PID_Limit_AWU/3(Ta)  "T2t_tiTaWastegateReqCorr"
  Logical Operator2/1 -> PID_Limit_AWU/6(initValue)
  Mpc_pManiFilt/1 -> Subtract/2
  Subtract1/1 -> T2t_facWasteGateRate/1
  T2t_rpmEngSpdpManiReq2facWastegateReqBase_MAP/1 -> Subtract1/1  "T2t_facWastegateReqBase"
  T2t_pManiReqSlow/1 -> Subtract/1, T2t_rpmEngSpdpManiReq2facWastegateReqBase_MAP/2
  Epm_rpmEngSpd/1 -> MinMax/1, T2t_rpmEngSpdpManiReq2facWastegateReqBase_MAP/1
  Constant9/1 -> PID_Limit_AWU/8(outMin)
  Constant8/1 -> PID_Limit_AWU/7(outMax)
  Constant7/1 -> PID_Limit_AWU/4(Kp)
  Constant6/1 -> PID_Limit_AWU/2(Tv)
  Subtract/1 -> PID_Limit_AWU/5(in)
  Constant5/1 -> PID_Limit_AWU/1(Tn)
  T2t_flgWasteGateControllerTrue/1 -> Logical Operator2/2
  Constant2/1 -> Logical Operator2/1
  PID_Limit_AWU/1(T2t_facWastegateReqCorr) -> Subtract1/2  "T2t_facWastegateReqCorr"

== system M160_lib/Functions/Tqs/EngSpdControl ==
  Epm_rpmEngSpd : Inport
  Egc_facEgas : Inport  Port=2
  Constan1 : Constant  Value=0.05  OutDataTypeStr=single
  Constan2 : Constant  Value=0.002  OutDataTypeStr=single
  Constan3 : Constant  Value=0.0  OutDataTypeStr=single
  Constant1 : Constant  Value=Tqs_flgIdleSpdCtrlEnable
  Constant2 : Constant  Value=Tqs_rpmEngSpdIdle
  Constant5 : Constant  Value=Tqs_tiTnIdleSpdCtrl
  Constant6 : Constant  Value=Tqs_tiTvIdleSpdCtrl
  Constant7 : Constant  Value=Tqs_facKIdleSpdCtrl
  Constant8 : Constant  Value=Tqs_tqIdleSpdCtrlMax
  Constant9 : Constant  Value=Tqs_tqIdleSpdCtrlMin
  Logical Operator2 : Logic  AllPortsSameDT=off  OutDataTypeStr=boolean
  PID_Limit_AWU : Subsystem
      mask Description: PID_Limit_AWU
      mask Display: image(imread('PID_Limit_AWU.jpg'))
  Relational Operator : RelationalOperator  Operator=<  OutDataTypeStr=boolean
  Subtract : Sum  Inputs=+-  OutDataTypeStr=Inherit: Same as first input
  Switch1 : Switch  Threshold=1
  Tqs_tqIdleSpdCtrlCorr : Outport
  wires:
  PID_Limit_AWU/1(Tqs_tqIdleSpdCtrlCorr) -> Switch1/3
  Constan1/1 -> Relational Operator/2
  Switch1/1 -> Tqs_tqIdleSpdCtrlCorr/1  "Tqs_tqIdleSpdCtrlCorr"
  Constant5/1 -> PID_Limit_AWU/1(Tn)
  Constan2/1 -> PID_Limit_AWU/3(Ta)
  Subtract/1 -> PID_Limit_AWU/5(in)
  Constant6/1 -> PID_Limit_AWU/2(Tv)
  Constant7/1 -> PID_Limit_AWU/4(Kp)
  Epm_rpmEngSpd/1 -> Subtract/2
  Constant2/1 -> Subtract/1
  Constant8/1 -> PID_Limit_AWU/7(outMax)
  Constant9/1 -> PID_Limit_AWU/8(outMin)
  Constan3/1 -> Switch1/1
  Constant1/1 -> Logical Operator2/1
  Relational Operator/1 -> Logical Operator2/2, PID_Limit_AWU/6(initValue)
  Egc_facEgas/1 -> Relational Operator/1
  Logical Operator2/1 -> Switch1/2

== system M160_lib/Sensors/Amc/G1_ADC_Input_Receive ==
  Data Type Conversion2 : DataTypeConversion  OutMin=0.0  OutMax=5.0  OutDataTypeStr=single
  Data Type Conversion3 : DataTypeConversion  OutMin=0.0  OutMax=1.0  OutDataTypeStr=boolean
  FlexECU_DevLib_FcnAPI_Wrapper_SFcn : S-Function  FunctionName=ehooks_medc17flex_devlib_basic_io_fcncall  Parameters=NoInputPorts, NoOutputPorts, InputPortDataTypes, OutputPortDataTypes, CFunctionArgTypes, CFunctionName, ChannelName  EnableBusSupport=off  mask{NoInputPorts=0, NoOutputPorts=2, InputPortDataTypes=, OutputPortDataTypes=uint8,int16, CFunctionArgTypes=ret,ref, CFunctionName=DevLib_Adc_Get, ChannelName=I_A_AN21}
      mask prompts: NoInputPorts "Number of input ports"; NoOutputPorts "Number of output ports"; InputPortDataTypes "Input port data types"; OutputPortDataTypes "Output port data types"; CFunctionArgTypes "C function argument types"; CFunctionName "C function name"; ChannelName "Channel (pin) name"
      mask Display: disp('EHOOKS FlexECU\nDevLib Wrapper\nS-Function')
  Gain : Gain  Gain=5/1023  OutDataTypeStr=Inherit: Same as input
  status : Outport
  uRaw : Outport  Port=2
  wires:
  Gain/1 -> uRaw/1
  Data Type Conversion2/1 -> Gain/1
  Data Type Conversion3/1 -> status/1
  FlexECU_DevLib_FcnAPI_Wrapper_SFcn/1 -> Data Type Conversion3/1
  FlexECU_DevLib_FcnAPI_Wrapper_SFcn/2 -> Data Type Conversion2/1

== system M160_lib/Sensors/Bvc/G1_ADC_Input_Receive ==
  Data Type Conversion2 : DataTypeConversion  OutMin=0.0  OutMax=5.0  OutDataTypeStr=single
  Data Type Conversion3 : DataTypeConversion  OutMin=0.0  OutMax=1.0  OutDataTypeStr=boolean
  FlexECU_DevLib_FcnAPI_Wrapper_SFcn : S-Function  FunctionName=ehooks_medc17flex_devlib_basic_io_fcncall  Parameters=NoInputPorts, NoOutputPorts, InputPortDataTypes, OutputPortDataTypes, CFunctionArgTypes, CFunctionName, ChannelName  EnableBusSupport=off  mask{NoInputPorts=0, NoOutputPorts=2, InputPortDataTypes=, OutputPortDataTypes=uint8,int16, CFunctionArgTypes=ret,ref, CFunctionName=DevLib_Adc_Get, ChannelName=I_A_AN16}
      mask prompts: NoInputPorts "Number of input ports"; NoOutputPorts "Number of output ports"; InputPortDataTypes "Input port data types"; OutputPortDataTypes "Output port data types"; CFunctionArgTypes "C function argument types"; CFunctionName "C function name"; ChannelName "Channel (pin) name"
      mask Display: disp('EHOOKS FlexECU\nDevLib Wrapper\nS-Function')
  Gain : Gain  Gain=5/1023  OutDataTypeStr=Inherit: Same as input
  status : Outport
  uRaw : Outport  Port=2
  wires:
  Gain/1 -> uRaw/1
  Data Type Conversion2/1 -> Gain/1
  Data Type Conversion3/1 -> status/1
  FlexECU_DevLib_FcnAPI_Wrapper_SFcn/1 -> Data Type Conversion3/1
  FlexECU_DevLib_FcnAPI_Wrapper_SFcn/2 -> Data Type Conversion2/1

== system M160_lib/Sensors/Cpc/Cpc_calc ==
  Epm_rpmEngSpd : Inport
  Cpc_pMani : Inport  Port=2
  Cpc_flgError : Inport  Port=3
  function : TriggerPort  TriggerType=function-call
  Accumulator : Subsystem
      mask Description: Accumulator
      mask Display: image(imread('Accumulator.jpg'))
  Constant1 : Constant  Value=0  OutDataTypeStr=single
  Constant2 : Constant  Value=0  OutDataTypeStr=single
  Constant6 : Constant  Value=30  OutDataTypeStr=single
  Counter : Subsystem
      mask Description: Counter
      mask Display: image(imread('Counter.jpg'))
  Divide : Product  Inputs=*/  OutDataTypeStr=single
  Logical Operator2 : Logic  Operator=NOT  AllPortsSameDT=off  OutDataTypeStr=boolean
  Logical Operator3 : Logic  AllPortsSameDT=off  OutDataTypeStr=boolean
  Relational Operator : RelationalOperator  Operator=>  OutDataTypeStr=boolean
  Relational Operator1 : RelationalOperator  Operator=>  OutDataTypeStr=boolean
  Switch : Switch  Threshold=1
  Switch1 : Switch  Threshold=1
  Cpc_pChargeFilt : Outport
  wires:
  Cpc_flgError/1 -> Logical Operator2/1
  Cpc_pMani/1 -> Switch1/1, Switch/3
  Logical Operator2/1 -> Logical Operator3/2
  Relational Operator/1 -> Logical Operator3/1
  Epm_rpmEngSpd/1 -> Relational Operator/1
  Constant6/1 -> Relational Operator/2
  Counter/1(Out1) -> Divide/2, Relational Operator1/1  "Cpc_nrValues"
  Constant1/1 -> Relational Operator1/2
  Relational Operator1/1 -> Switch/2
  Constant2/1 -> Accumulator/2(initValue), Switch1/3
  Accumulator/1(Out2) -> Divide/1  "Cpc_pAccu"
  Switch/1 -> Cpc_pChargeFilt/1  "Cpc_pChargeFilt"
  Divide/1 -> Switch/1
  Logical Operator3/1 -> Switch1/2
  Switch1/1 -> Accumulator/1(in), Counter/1(in)

== system M160_lib/Sensors/Cpc/Cpc_get ==
  Mtc_atMani : Inport
  function : TriggerPort  TriggerType=function-call
  Constant3 : Constant  Value=0  OutDataTypeStr=boolean
  Constant4 : Constant  Value=Cpc_flgPChargeOverride
  Cpc_atManiTmp2facPresCorr_CUR : Lookup_n-D  NumberOfTableDimensions=1  BreakpointsForDimension1=Cpc_atManiTmp2facPresCorr_CUR_x  BreakpointsForDimension1DataTypeStr=Inherit: Inherit from 'Breakpoint data'  Table=Cpc_atManiTmp2facPresCorr_CUR_y  TableDataTypeStr=Inherit: Inherit from 'Table data'  ExtrapMethod=Clip  OutDataTypeStr=Inherit: Inherit from 'Table data'  InputSameDT=on
  Cpc_uSens2pManiBase_CUR : Lookup_n-D  NumberOfTableDimensions=1  BreakpointsForDimension1=Cpc_uSens2pManiBase_CUR_x  BreakpointsForDimension1DataTypeStr=Inherit: Inherit from 'Breakpoint data'  Table=Cpc_uSens2pManiBase_CUR_y  TableDataTypeStr=Inherit: Inherit from 'Table data'  ExtrapMethod=Clip  OutDataTypeStr=Inherit: Inherit from 'Table data'  InputSameDT=on
  G1_ADC_Input_Receive : Subsystem  LoadFcn=ehooks_medc17flex_devlib_io_block('load');  InitFcn=ehooks_medc17flex_devlib_io_block('init');  StartFcn=ehooks_medc17flex_devlib_io_block('start');  StopFcn=ehooks_medc17flex_devlib_io_block('stop');  ClipboardFcn=ehooks_medc17flex_devlib_io_block('clipboard', 0); % Second argument just needed to indicate null block. See callback handler.  mask{ChannelName=I_A_AN05}
      mask prompts: ChannelName "Channel name"
      mask init:
      | ehooks_medc17flex_devlib_io_block('mask_init');
      settings: AttributesFormatString=Channel name: '%<ChannelName>'  CopyFcn=ehooks_medc17flex_devlib_io_block('copy');  DeleteFcn=ehooks_medc17flex_devlib_io_block('delete');  UndoDeleteFcn=ehooks_medc17flex_devlib_io_block('undo_delete');  ModelCloseFcn=ehooks_medc17flex_devlib_io_block('model_close');  PreSaveFcn=ehooks_medc17flex_devlib_io_block('pre_save');  PostSaveFcn=ehooks_medc17flex_devlib_io_block('post_save');  NameChangeFcn=ehooks_medc17flex_devlib_io_block('name_change');  DestroyFcn=ehooks_medc17flex_devlib_io_block('destroy', 0); % Second argument just needed to indicate null block. See callback handler.  OpenFcn=ehooks_medc17flex_devlib_io_block('open');  CloseFcn=ehooks_medc17flex_devlib_io_block('close');  ParentCloseFcn=ehooks_medc17flex_devlib_io_block('parent_close');  MoveFcn=ehooks_medc17flex_devlib_io_block('move');
      mask StyleString: popup(<empty>|I_A_AN01|I_A_AN02|I_A_AN03|I_A_AN05|I_A_AN06|I_A_AN07|I_A_AN08|I_A_AN10|I_A_AN11|I_A_AN12|I_A_AN13|I_A_AN14|I_A_AN15|I_A_AN16|I_A_AN17|I_A_AN18|I_A_AN19|I_A_AN20|I_A_AN21|I_A_AN23|I_A_AN32|I_A_AN35|I_A_AN36|I_A_AN37|I_A_AN39|I_A_AN100|I_A_AN101|I_A_AN103|I_A_AN104|I_A_AN105|I_A_AN106)
      mask Display: image(imread('Input_Analog.jpg'))
  Interval Test : simulink/Logic and Bit Operations/Interval Test  IntervalClosedRight=on  uplimit=Mpc_uSensMaxValid  IntervalClosedLeft=on  lowlimit=Mpc_uSensMinValid  OutDataTypeStr=boolean
  Logical Operator : Logic  Operator=NOT  AllPortsSameDT=off  OutDataTypeStr=boolean
  Logical Operator1 : Logic  Operator=NOT  AllPortsSameDT=off  OutDataTypeStr=boolean
  Logical Operator4 : Logic  Operator=OR  AllPortsSameDT=off  OutDataTypeStr=boolean
  Product : Product  OutDataTypeStr=Inherit: Same as first input
  Switch2 : Switch  Threshold=1
  Cpc_flgError : Outport
  Cpc_pMani : Outport  Port=2
  wires:
  Cpc_atManiTmp2facPresCorr_CUR/1 -> Product/2
  Cpc_uSens2pManiBase_CUR/1 -> Product/1
  Mtc_atMani/1 -> Cpc_atManiTmp2facPresCorr_CUR/1
  Product/1 -> Cpc_pMani/1  "Cpc_pMani"
  G1_ADC_Input_Receive/1(status) -> Logical Operator/1  "Cpc_stIOError"
  G1_ADC_Input_Receive/2(uRaw) -> Cpc_uSens2pManiBase_CUR/1, Interval Test/1  "Cpc_uSens"
  Interval Test/1 -> Logical Operator1/1
  Logical Operator/1 -> Logical Operator4/1
  Logical Operator1/1 -> Logical Operator4/2
  Switch2/1 -> Cpc_flgError/1  "Cpc_flgError"
  Logical Operator4/1 -> Switch2/3
  Constant3/1 -> Switch2/1
  Constant4/1 -> Switch2/2

== system M160_lib/Sensors/Cpc/Cpc_pCharge_calc ==
  ECU_FcnCallTrigger_Source_DownStream : Subsystem  TreatAsAtomicUnit=on
  TriggerOut : Outport
  wires:
  ECU_FcnCallTrigger_Source_DownStream/1(TriggerOut) -> TriggerOut/1

== system M160_lib/Sensors/Cpc/Cpc_pCharge_get ==
  ECU_FcnCallTrigger_Source_DownStream : Subsystem  TreatAsAtomicUnit=on
  TriggerOut : Outport
  wires:
  ECU_FcnCallTrigger_Source_DownStream/1(TriggerOut) -> TriggerOut/1

== system M160_lib/Sensors/Ctc/G1_ADC_Input_Receive ==
  Data Type Conversion2 : DataTypeConversion  OutMin=0.0  OutMax=5.0  OutDataTypeStr=single
  Data Type Conversion3 : DataTypeConversion  OutMin=0.0  OutMax=1.0  OutDataTypeStr=boolean
  FlexECU_DevLib_FcnAPI_Wrapper_SFcn : S-Function  FunctionName=ehooks_medc17flex_devlib_basic_io_fcncall  Parameters=NoInputPorts, NoOutputPorts, InputPortDataTypes, OutputPortDataTypes, CFunctionArgTypes, CFunctionName, ChannelName  EnableBusSupport=off  mask{NoInputPorts=0, NoOutputPorts=2, InputPortDataTypes=, OutputPortDataTypes=uint8,int16, CFunctionArgTypes=ret,ref, CFunctionName=DevLib_Adc_Get, ChannelName=I_A_AN10}
      mask prompts: NoInputPorts "Number of input ports"; NoOutputPorts "Number of output ports"; InputPortDataTypes "Input port data types"; OutputPortDataTypes "Output port data types"; CFunctionArgTypes "C function argument types"; CFunctionName "C function name"; ChannelName "Channel (pin) name"
      mask Display: disp('EHOOKS FlexECU\nDevLib Wrapper\nS-Function')
  Gain : Gain  Gain=5/1023  OutDataTypeStr=Inherit: Same as input
  status : Outport
  uRaw : Outport  Port=2
  wires:
  FlexECU_DevLib_FcnAPI_Wrapper_SFcn/2 -> Data Type Conversion2/1
  FlexECU_DevLib_FcnAPI_Wrapper_SFcn/1 -> Data Type Conversion3/1
  Data Type Conversion3/1 -> status/1
  Data Type Conversion2/1 -> Gain/1
  Gain/1 -> uRaw/1
